simulink model "PMSM_model"  (R2014b)
settings: Solver=ode45  StartTime=0.0  StopTime=10.0  RelTol=1e-3
undefined symbols (not defined in the file or in its folder): Ll
settings Model: CovSFcnEnable=on  Creator=Lei  LastModifiedBy=Lei
settings DataIOCC: SignalLoggingSaveFormat=ModelDataLogs  SignalLoggingName=sigsOut
settings DebuggingCC: SaveWithParameterizedLinksMsg=none  UnderspecifiedInitializationDetection=Classic  MergeDetectMultiDrivingBlocksExec=none  SignalResolutionControl=TryResolveAllWithWarning  SolverPrmCheckMsg=none  MultiTaskDSMMsg=warning  MultiTaskCondExecSysMsg=none  FrameProcessingCompatibilityMsg=error  StrictBusMsg=None
settings HardwareCC: TargetUnknown=on
settings GRTTargetCC: CombineOutputUpdateFcns=off  GRTInterface=on

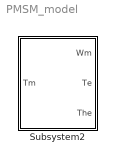
== system PMSM_model ==
  Subsystem2 : Subsystem

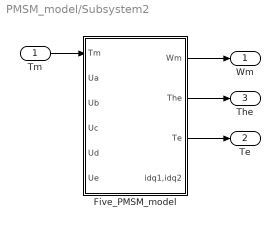
== system PMSM_model/Subsystem2 ==
  Tm : Inport
  Five_PMSM_model : Subsystem  mask{Ld=0, Lq=0, R=0, Pn=0, flux=0, B=0, J=0}
      mask prompts: Ld "d-Inductances(Ld)"; Lq "q-Inductances(Lq)"; R "resistance(R)"; Pn "pole pairs(Pn)"; flux "Flux linkage(flux)"; B "viscous damping(B)"; J "Inertia(J)"
  Wm : Outport
  Te : Outport  Port=2
  The : Outport  Port=3
  wires:
  Tm/1 -> Five_PMSM_model/1(Tm)
  Five_PMSM_model/1(Wm) -> Wm/1
  Five_PMSM_model/3(Te) -> Te/1
  Five_PMSM_model/2(The) -> The/1

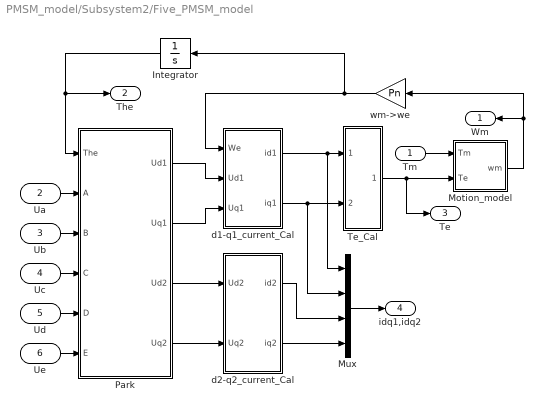
== system PMSM_model/Subsystem2/Five_PMSM_model ==
  Tm : Inport
  Ua : Inport  Port=2
  Ub : Inport  Port=3
  Uc : Inport  Port=4
  Ud : Inport  Port=5
  Ue : Inport  Port=6
  Integrator : Integrator
  Motion_model : Subsystem
  Mux : Mux
  Park : Subsystem
  Te_Cal : Subsystem
  d1-q1_current_Cal : Subsystem
  d2-q2_current_Cal : Subsystem
  wm->we : Gain  Gain=Pn  SaturateOnIntegerOverflow=on  OutDataTypeStr=Inherit: Same as input  ParamDataTypeStr=Inherit: Same as input
  Wm : Outport
  The : Outport  Port=2
  Te : Outport  Port=3
  idq1,idq2 : Outport  Port=4
  wires:
  d1-q1_current_Cal/1(id1) -> Mux/1, Te_Cal/1(id1)
  d1-q1_current_Cal/2(iq1) -> Mux/2, Te_Cal/2(iq1)
  wm->we/1 -> Integrator/1, d1-q1_current_Cal/1(We)
  Motion_model/1(wm) -> Wm/1, wm->we/1
  Te_Cal/1(Te) -> Te/1, Motion_model/2(Te)
  Tm/1 -> Motion_model/1(Tm)
  Ub/1 -> Park/3(B)
  Uc/1 -> Park/4(C)
  Ua/1 -> Park/2(A)
  Ud/1 -> Park/5(D)
  Ue/1 -> Park/6(E)
  Park/1("Ud1 ") -> d1-q1_current_Cal/2(Ud1)
  Park/2(Uq1) -> d1-q1_current_Cal/3(Uq1)
  Integrator/1 -> The/1, Park/1(The)
  Park/4(Uq2) -> d2-q2_current_Cal/2(Uq2)
  Park/3(Ud2) -> d2-q2_current_Cal/1(Ud2)
  Mux/1 -> idq1,idq2/1
  d2-q2_current_Cal/1(id2) -> Mux/3
  d2-q2_current_Cal/2(iq2) -> Mux/4

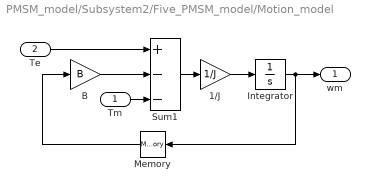
== system PMSM_model/Subsystem2/Five_PMSM_model/Motion_model ==
  Tm : Inport
  Te : Inport  Port=2
  1/J : Gain  Gain=1/J  SaturateOnIntegerOverflow=on  OutDataTypeStr=Inherit: Same as input  ParamDataTypeStr=Inherit: Same as input
  B : Gain  Gain=B  SaturateOnIntegerOverflow=on  OutDataTypeStr=Inherit: Same as input  ParamDataTypeStr=Inherit: Same as input
  Integrator : Integrator
  Memory : Memory
  Sum1 : Sum  Inputs=+--  SaturateOnIntegerOverflow=on
  wm : Outport
  wires:
  Tm/1 -> Sum1/3
  Sum1/1 -> 1/J/1
  B/1 -> Sum1/2
  1/J/1 -> Integrator/1
  Te/1 -> Sum1/1
  Integrator/1 -> Memory/1, wm/1
  Memory/1 -> B/1

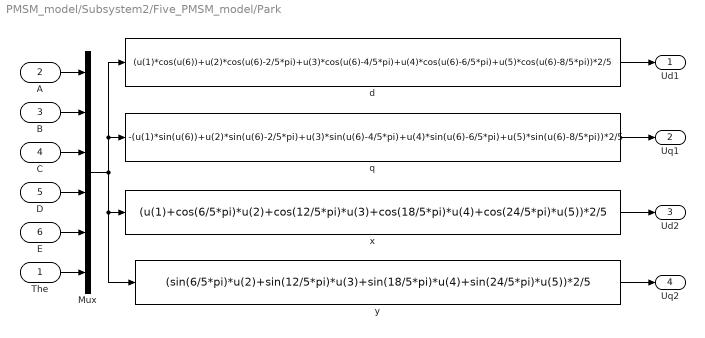
== system PMSM_model/Subsystem2/Five_PMSM_model/Park ==
  The : Inport
  A : Inport  Port=2
  B : Inport  Port=3
  C : Inport  Port=4
  D : Inport  Port=5
  E : Inport  Port=6
  Mux : Mux  Inputs=6
  d : Fcn  Expr=(u(1)*cos(u(6))+u(2)*cos(u(6)-2/5*pi)+u(3)*cos(u(6)-4/5*pi)+u(4)*cos(u(6)-6/5*pi)+u(5)*cos(u(6)-8/5*pi))*2/5
  q : Fcn  Expr=-(u(1)*sin(u(6))+u(2)*sin(u(6)-2/5*pi)+u(3)*sin(u(6)-4/5*pi)+u(4)*sin(u(6)-6/5*pi)+u(5)*sin(u(6)-8/5*pi))*2/5
  "x " : Fcn  Expr=(u(1)+cos(6/5*pi)*u(2)+cos(12/5*pi)*u(3)+cos(18/5*pi)*u(4)+cos(24/5*pi)*u(5))*2/5
  "y " : Fcn  Expr=(sin(6/5*pi)*u(2)+sin(12/5*pi)*u(3)+sin(18/5*pi)*u(4)+sin(24/5*pi)*u(5))*2/5
  "Ud1 " : Outport
  Uq1 : Outport  Port=2
  Ud2 : Outport  Port=3
  Uq2 : Outport  Port=4
  wires:
  d/1 -> "Ud1 "/1
  B/1 -> Mux/2
  C/1 -> Mux/3
  A/1 -> Mux/1
  D/1 -> Mux/4
  E/1 -> Mux/5
  The/1 -> Mux/6
  Mux/1 -> q/1, d/1, "y "/1, "x "/1
  q/1 -> Uq1/1
  "x "/1 -> Ud2/1
  "y "/1 -> Uq2/1

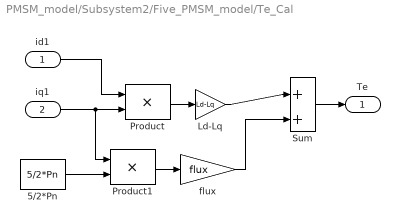
== system PMSM_model/Subsystem2/Five_PMSM_model/Te_Cal ==
  id1 : Inport
  iq1 : Inport  Port=2
  5/2*Pn : Constant  Value=5/2*Pn
  Ld-Lq : Gain  Gain=Ld-Lq  SaturateOnIntegerOverflow=on  OutDataTypeStr=Inherit: Same as input  ParamDataTypeStr=Inherit: Same as input
  Product : Product  SaturateOnIntegerOverflow=on  OutDataTypeStr=Inherit: Same as first input
  Product1 : Product  SaturateOnIntegerOverflow=on  OutDataTypeStr=Inherit: Same as first input
  Sum : Sum  Inputs=|++  SaturateOnIntegerOverflow=on
  flux : Gain  Gain=flux  SaturateOnIntegerOverflow=on  OutDataTypeStr=Inherit: Same as input  ParamDataTypeStr=Inherit: Same as input
  Te : Outport
  wires:
  iq1/1 -> Product/2, Product1/1
  id1/1 -> Product/1
  5/2*Pn/1 -> Product1/2
  Ld-Lq/1 -> Sum/1
  Product/1 -> Ld-Lq/1
  flux/1 -> Sum/2
  Product1/1 -> flux/1
  Sum/1 -> Te/1

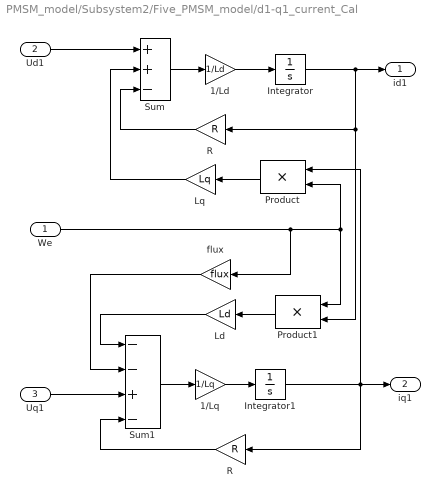
== system PMSM_model/Subsystem2/Five_PMSM_model/d1-q1_current_Cal ==
  We : Inport
  Ud1 : Inport  Port=2
  Uq1 : Inport  Port=3
  1/Ld : Gain  Gain=1/Ld  SaturateOnIntegerOverflow=on  OutDataTypeStr=Inherit: Same as input  ParamDataTypeStr=Inherit: Same as input
  1/Lq : Gain  Gain=1/Lq  SaturateOnIntegerOverflow=on  OutDataTypeStr=Inherit: Same as input  ParamDataTypeStr=Inherit: Same as input
  Integrator : Integrator  InitialCondition=0.01
  Integrator1 : Integrator
  Ld : Gain  Gain=Ld  SaturateOnIntegerOverflow=on  OutDataTypeStr=Inherit: Same as input  ParamDataTypeStr=Inherit: Same as input
  Lq : Gain  Gain=Lq  SaturateOnIntegerOverflow=on  OutDataTypeStr=Inherit: Same as input  ParamDataTypeStr=Inherit: Same as input
  Product : Product  SaturateOnIntegerOverflow=on  OutDataTypeStr=Inherit: Same as first input
  Product1 : Product  SaturateOnIntegerOverflow=on  OutDataTypeStr=Inherit: Same as first input
  R : Gain  Gain=R  SaturateOnIntegerOverflow=on  OutDataTypeStr=Inherit: Same as input  ParamDataTypeStr=Inherit: Same as input
  "R " : Gain  Gain=R  SaturateOnIntegerOverflow=on  OutDataTypeStr=Inherit: Same as input  ParamDataTypeStr=Inherit: Same as input
  Sum : Sum  Inputs=++-  SaturateOnIntegerOverflow=on
  Sum1 : Sum  Inputs=--+-  SaturateOnIntegerOverflow=on
  flux : Gain  Gain=flux  SaturateOnIntegerOverflow=on  OutDataTypeStr=Inherit: Same as input  ParamDataTypeStr=Inherit: Same as input
  id1 : Outport
  iq1 : Outport  Port=2
  wires:
  Ud1/1 -> Sum/1
  Sum/1 -> 1/Ld/1
  1/Ld/1 -> Integrator/1
  Integrator/1 -> Product1/2, R/1, id1/1
  Product/1 -> Lq/1
  Lq/1 -> Sum/2
  We/1 -> Product/2, Product1/1, flux/1
  R/1 -> Sum/3
  "R "/1 -> Sum1/4
  1/Lq/1 -> Integrator1/1
  Sum1/1 -> 1/Lq/1
  Integrator1/1 -> "R "/1, Product/1, iq1/1
  Product1/1 -> Ld/1
  Ld/1 -> Sum1/1
  Uq1/1 -> Sum1/3
  flux/1 -> Sum1/2

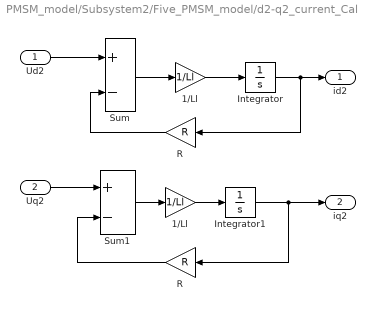
== system PMSM_model/Subsystem2/Five_PMSM_model/d2-q2_current_Cal ==
  Ud2 : Inport
  Uq2 : Inport  Port=2
  1/Ll : Gain  Gain=1/Ll  SaturateOnIntegerOverflow=on  OutDataTypeStr=Inherit: Same as input  ParamDataTypeStr=Inherit: Same as input
  "1/Ll " : Gain  Gain=1/Ll  SaturateOnIntegerOverflow=on  OutDataTypeStr=Inherit: Same as input  ParamDataTypeStr=Inherit: Same as input
  Integrator : Integrator  InitialCondition=0.01
  Integrator1 : Integrator
  R : Gain  Gain=R  SaturateOnIntegerOverflow=on  OutDataTypeStr=Inherit: Same as input  ParamDataTypeStr=Inherit: Same as input
  "R " : Gain  Gain=R  SaturateOnIntegerOverflow=on  OutDataTypeStr=Inherit: Same as input  ParamDataTypeStr=Inherit: Same as input
  Sum : Sum  Inputs=+-  SaturateOnIntegerOverflow=on
  Sum1 : Sum  Inputs=+-  SaturateOnIntegerOverflow=on
  id2 : Outport
  iq2 : Outport  Port=2
  wires:
  Uq2/1 -> Sum1/1
  Integrator1/1 -> iq2/1, "R "/1
  Sum1/1 -> 1/Ll/1
  1/Ll/1 -> Integrator1/1
  "R "/1 -> Sum1/2
  R/1 -> Sum/2
  Integrator/1 -> id2/1, R/1
  "1/Ll "/1 -> Integrator/1
  Sum/1 -> "1/Ll "/1
  Ud2/1 -> Sum/1
